simulink model "dc_microgrid"  (R2014a)
settings: Solver=ode45  StartTime=0.0  StopTime=Tmax  RelTol=1e-3
values from neighbouring files (symbols this model uses):
  a1v1 = Pmc*a1xpi1    [parameters_dcmicrogrid.m]
  a1v2 = Pmc*a1xpi2    [parameters_dcmicrogrid.m]
  a1xmc1 = a3    [parameters_dcmicrogrid.m]
  a1xmc2 = a3    [parameters_dcmicrogrid.m]
  a1xpi1 = Imc*c3    [parameters_dcmicrogrid.m]
  a1xpi2 = Imc*c3    [parameters_dcmicrogrid.m]
  a2v1 = Pmc*a2xpi1    [parameters_dcmicrogrid.m]
  a2v2 = Pmc*a2xpi2    [parameters_dcmicrogrid.m]
  a2xmc1 = C(1,2)*P(1,1)*c1/Imax(1)    [parameters_dcmicrogrid.m]
  a2xmc2 = C(2,1)*P(2,2)*c1/Imax(2)    [parameters_dcmicrogrid.m]
  a2xpi1 = Imc*c2    [parameters_dcmicrogrid.m]
  a2xpi2 = Imc*c2    [parameters_dcmicrogrid.m]
  a3xmc1 = C(1,2)*P(1,1)*c1/Imax(1) + RD(1,1)*c1    [parameters_dcmicrogrid.m]
  a3xmc2 = C(1,2)*P(2,2)*c1/Imax(2) + RD(2,2)*c1    [parameters_dcmicrogrid.m]
  axi1 = C(1,2)*I(1,1)*c1/Imax(1)    [parameters_dcmicrogrid.m]
  axi2 = C(2,1)*I(2,2)*c1/Imax(2)    [parameters_dcmicrogrid.m]
  C1 = 2.2e-3    (= 0.0022)    [parameters_dcmicrogrid.m]
  C2 = 2.2e-3    (= 0.0022)    [parameters_dcmicrogrid.m]
  iL1_0 = 4.5    [parameters_dcmicrogrid.m]
  iL2_0 = 4.5    [parameters_dcmicrogrid.m]
  L1 = 2.65e-3    (= 0.00265)    [parameters_dcmicrogrid.m]
  L2 = 2.65e-3    (= 0.00265)    [parameters_dcmicrogrid.m]
  R1 = 20    [parameters_dcmicrogrid.m]
  R2 = 20    [parameters_dcmicrogrid.m]
  Req = R1*R2/(R1+R2)    (= 10)    [parameters_dcmicrogrid.m]
  rL1 = 520e-3    (= 0.52)    [parameters_dcmicrogrid.m]
  rL2 = 520e-3    (= 0.52)    [parameters_dcmicrogrid.m]
  rs1 = 200e-3    (= 0.2)    [parameters_dcmicrogrid.m]
  rs2 = 200e-3    (= 0.2)    [parameters_dcmicrogrid.m]
  T1 = 1/Fs    (= 6.66666666667e-05)    [parameters_dcmicrogrid.m]
  T2 = 1/Fs    (= 6.66666666667e-05)    [parameters_dcmicrogrid.m]
  t_0 = 0    [parameters_dcmicrogrid.m]
  vC1_0 = 48.02    [parameters_dcmicrogrid.m]
  vC2_0 = 48.02    [parameters_dcmicrogrid.m]
  Vin1 = Vin(1)    [parameters_dcmicrogrid.m]
  Vin2 = Vin(2)    [parameters_dcmicrogrid.m]
  Vref1 = Vref(1)    [parameters_dcmicrogrid.m]
  Vref2 = Vref(2)    [parameters_dcmicrogrid.m]
  xi1_0 = 0.01915    [parameters_dcmicrogrid.m]
  xi2_0 = 0.01915    [parameters_dcmicrogrid.m]
  xmc1_0 = 2.401    [parameters_dcmicrogrid.m]
  xmc2_0 = 2.401    [parameters_dcmicrogrid.m]
  xpi1_0 = 0.51    [parameters_dcmicrogrid.m]
  xpi2_0 = 0.51    [parameters_dcmicrogrid.m]
  xpu1_0 = 0.01275    [parameters_dcmicrogrid.m]
  xpu2_0 = 0.01275    [parameters_dcmicrogrid.m]
  xvo1_0 = 0.0103    [parameters_dcmicrogrid.m]
  xvo2_0 = 0.0103    [parameters_dcmicrogrid.m]
undefined symbols (not defined in the file or in its folder): a1, a2, b1, b2, c1, c2, d1, d2
settings Model: Creator=OmarAli  LastModifiedBy=OmarAli
settings DataIOCC: LimitDataPoints=off
settings DebuggingCC: MergeDetectMultiDrivingBlocksExec=error  FrameProcessingCompatibilityMsg=error

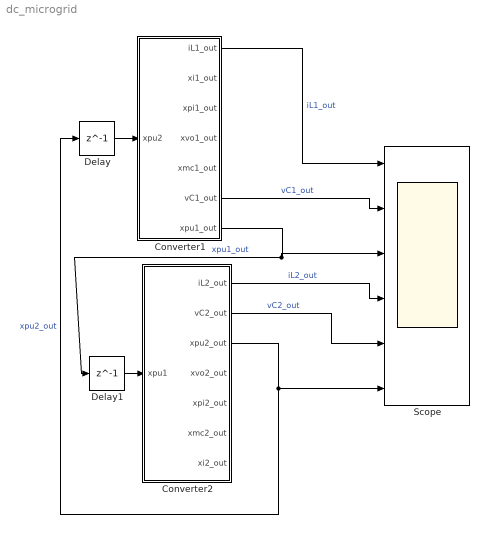
== system dc_microgrid ==
  Converter1 : Stateflow chart  TreatAsAtomicUnit=on
  Converter2 : Stateflow chart  TreatAsAtomicUnit=on
  Delay : Delay  DelayLength=1  InitialCondition=0  SampleTime=1/60000
  Delay1 : Delay  DelayLength=1  InitialCondition=0  SampleTime=1/60000
  Scope : Scope  NumInputPorts=6
      settings: ShowLegends=on  YMin=-5~-5~-5~-5~-5~-5  YMax=5~5~5~5~5~5
  wires:
  Converter1/7(xpu1_out) -> Scope/3, Delay1/1  "xpu1_out"
  Converter2/3(xpu2_out) -> Scope/6, Delay/1  "xpu2_out"
  Delay/1 -> Converter1/1(xpu2)
  Delay1/1 -> Converter2/1(xpu1)
  Converter1/1(iL1_out) -> Scope/1  "iL1_out"
  Converter1/6(vC1_out) -> Scope/2  "vC1_out"
  Converter2/1(iL2_out) -> Scope/4  "iL2_out"
  Converter2/2(vC2_out) -> Scope/5  "vC2_out"

== stateflow chart dc_microgrid/Converter2 ==
  settings: updateMethod=CONTINUOUS
  state close2
    du:
    iL2_dot = (1/L2)*(-1*(rs2+rL2)*iL2+Vin2 - vC2);
    vC2_dot = (1/C2)*(iL2 - vC2/Req);
    xpu2_dot = a1*xpu2 + b1*iL2;
    xi2_dot = axi2*(xpu1 - xpu2);
    xmc2_dot = a1xmc2*xmc2 + a2xmc2*xpu1 - a3xmc2*xpu2 + xi2+ Vref2;
    xvo2_dot = a2*xvo2 + b2*vC2;
    xpi2_dot = a1xpi2*xmc2 - a2xpi2*xvo2;
    t_dot = 1;
    iL2_out = iL2;
    vC2_out = vC2;
    xpu2_out = xpu2;
    xi2_out = xi2;
    xmc2_out =xmc2;
    xvo2_out = xvo2;
    xpi2_out = xpi2;
  state open2
    du:
    iL2_dot = (1/L2)*(-rL2*iL2 - vC2);
    vC2_dot = (1/C2)*(iL2 - vC2/Req);
    xpu2_dot = a1*xpu2 + b1*iL2;
    xi2_dot = axi2*(xpu1 - xpu2);
    xmc2_dot = a1xmc2*xmc2 + a2xmc2*xpu1 - a3xmc2*xpu2 + xi2+ Vref2;
    xvo2_dot = a2*xvo2 + b2*vC2;
    xpi2_dot = a1xpi2*xmc2 - a2xpi2*xvo2;
    t_dot = 1;
    iL2_out = iL2;
    vC2_out = vC2;
    xpu2_out = xpu2;
    xi2_out = xi2;
    xmc2_out =xmc2;
    xvo2_out = xvo2;
    xpi2_out = xpi2;
  state dcm2
    du:
    iL2_dot = 0;
    vC2_dot = - vC2/(Req*C2);
    xpu2_dot = a1*xpu2 + b1*iL2;
    xi2_dot = axi2*(xpu1 - xpu2);
    xmc2_dot = a1xmc2*xmc2 + a2xmc2*xpu1 - a3xmc2*xpu2 + xi2+ Vref2;
    xvo2_dot = a2*xvo2 + b2*vC2;
    xpi2_dot = a1xpi2*xmc2 - a2xpi2*xvo2;
    t_dot = 1;
    iL2_out = iL2;
    vC2_out = vC2;
    xpu2_out = xpu2;
    xi2_out = xi2;
    xmc2_out =xmc2;
    xvo2_out = xvo2;
    xpi2_out = xpi2;
  (default) -> close2 : {iL2 = iL2_0;
      | vC2 = vC2_0;
      | xpu2 = xpu2_0;
      | xi2 = xi2_0;
      | xmc2 = xmc2_0;
      | xvo2 = xvo2_0;
      | xpi2 = xpi2_0;
      | t = t_0;}
  close2 -> open2 : [(a1v2*xmc2 - a2v2*xvo2 + xpi2) -  t/T2<= 0]
  open2 -> close2 [order 2] : [t >= T2]
      | {t = 0;}
  dcm2 -> close2 : [t >= T2]
      | {t = 0;}
  open2 -> dcm2 [order 1] : [iL2 <= 0]
  data: rs2 parameter double; Vref2 parameter double; Vin2 parameter double; rL2 parameter double; iL2_out output double; t local; iL2 local; vC2 local; xi2 local; xvo2 local; xpu2 local; xmc2 local; xpi2 local; T2 parameter double; L2 parameter double; C2 parameter double; R2 parameter double; vC2_out output double; xpu2_out output double; xvo2_out output double; xpi2_out output double; xmc2_out output double; xi2_out output double; xpu1 input double; a1 parameter double; a2 parameter double; b1 parameter double; b2 parameter double; c1 parameter double; c2 parameter double; d1 parameter double; d2 parameter double; axi2 parameter double; a1xmc2 parameter double; a2xmc2 parameter double; a3xmc2 parameter double; a1xpi2 parameter double; a2xpi2 parameter double; a1v2 parameter double; a2v2 parameter double; Req parameter double; iL2_0 parameter; t_0 parameter; xpu2_0 parameter; xmc2_0 parameter; xvo2_0 parameter; xpi2_0 parameter; vC2_0 parameter; xi2_0 parameter
  data t settings: updateMethod=SF_CONTINUOUS_TIME_DATA
  data iL2 settings: updateMethod=SF_CONTINUOUS_TIME_DATA
  data vC2 settings: updateMethod=SF_CONTINUOUS_TIME_DATA
  data xi2 settings: updateMethod=SF_CONTINUOUS_TIME_DATA
  data xvo2 settings: updateMethod=SF_CONTINUOUS_TIME_DATA
  data xpu2 settings: updateMethod=SF_CONTINUOUS_TIME_DATA
  data xmc2 settings: updateMethod=SF_CONTINUOUS_TIME_DATA
  data xpi2 settings: updateMethod=SF_CONTINUOUS_TIME_DATA

== stateflow chart dc_microgrid/Converter1 ==
  settings: updateMethod=CONTINUOUS
  state close1
    du:
    iL1_dot = (1/L1)*(-1*(rs1+rL1)*iL1+Vin1 - vC1);
    vC1_dot = (1/C1)*(iL1 - vC1/Req);
    xpu1_dot = a1*xpu1 + b1*iL1;
    xi1_dot = axi1*(xpu2 - xpu1);
    xmc1_dot = a1xmc1*xmc1 + a2xmc1*xpu2  - a3xmc1*xpu1 + xi1+ Vref1;
    xvo1_dot = a2*xvo1 + b2*vC1;
    xpi1_dot = a1xpi1*xmc1 - a2xpi1*xvo1;
    t_dot = 1;
    iL1_out = iL1;
    vC1_out = vC1;
    xpu1_out = xpu1;
    xi1_out = xi1;
    xmc1_out =xmc1;
    xvo1_out = xvo1;
    xpi1_out = xpi1;
  state open1
    du:
    iL1_dot = (1/L1)*(-rL1*iL1 - vC1);
    vC1_dot = (1/C1)*(iL1 - vC1/Req);
    xpu1_dot = a1*xpu1 + b1*iL1;
    xi1_dot = axi1*(xpu2 - xpu1);
    xmc1_dot = a1xmc1*xmc1 + a2xmc1*xpu2  - a3xmc1*xpu1 + xi1+ Vref1;
    xvo1_dot = a2*xvo1 + b2*vC1;
    xpi1_dot = a1xpi1*xmc1 - a2xpi1*xvo1;
    t_dot = 1;
    iL1_out = iL1;
    vC1_out = vC1;
    xpu1_out = xpu1;
    xi1_out = xi1;
    xmc1_out =xmc1;
    xvo1_out = xvo1;
    xpi1_out = xpi1;
  state dcm1
    du:
    iL1_dot = 0;
    vC1_dot = - vC1/(Req*C1);
    xpu1_dot = a1*xpu1 + b1*iL1;
    xi1_dot = axi1*(xpu2 - xpu1);
    xmc1_dot = a1xmc1*xmc1 + a2xmc1*xpu2  - a3xmc1*xpu1 + xi1+ Vref1;
    xvo1_dot = a2*xvo1 + b2*vC1;
    xpi1_dot = a1xpi1*xmc1 - a2xpi1*xvo1;
    t_dot = 1;
    iL1_out = iL1;
    vC1_out = vC1;
    xpu1_out = xpu1;
    xi1_out = xi1;
    xmc1_out =xmc1;
    xvo1_out = xvo1;
    xpi1_out = xpi1;
  (default) -> close1 : {iL1 = iL1_0;
      | vC1 = vC1_0;
      | xpu1 = xpu1_0;
      | xi1 = xi1_0;
      | xmc1 = xmc1_0;
      | xvo1 = xvo1_0;
      | xpi1 = xpi1_0;
      | t = t_0;}
  close1 -> open1 : [(a1v1*xmc1 - a2v1*xvo1 + xpi1) -  t/T1 <= 0]
  open1 -> close1 [order 2] : [t >= T1]
      | {t = 0;}
  dcm1 -> close1 : [t >= T1]
      | {t = 0;}
  open1 -> dcm1 [order 1] : [iL1 <= 0]
  data: rL1 parameter double; Vin1 parameter double; rs1 parameter double; Vref1 parameter double; iL1_out output double; xpu1 local; iL1 local; xmc1 local; vC1 local; xpi1 local; xvo1 local; xi1 local; t local; C1 parameter double; R1 parameter double; L1 parameter double; T1 parameter double; xi1_out output double; xpi1_out output double; xvo1_out output double; xmc1_out output double; vC1_out output double; xpu1_out output double; xpu2 input double; a1 parameter double; a2 parameter double; b1 parameter double; b2 parameter double; c1 parameter double; c2 parameter double; d1 parameter double; d2 parameter double; axi1 parameter double; a1xmc1 parameter double; a2xmc1 parameter double; a3xmc1 parameter double; a1xpi1 parameter double; a2xpi1 parameter double; a1v1 parameter double; a2v1 parameter double; Req parameter double; xvo1_0 parameter; xpi1_0 parameter; xmc1_0 parameter; xi1_0 parameter; iL1_0 parameter; vC1_0 parameter; xpu1_0 parameter; t_0 parameter
  data xpu1 settings: updateMethod=SF_CONTINUOUS_TIME_DATA
  data iL1 settings: updateMethod=SF_CONTINUOUS_TIME_DATA
  data xmc1 settings: updateMethod=SF_CONTINUOUS_TIME_DATA
  data vC1 settings: updateMethod=SF_CONTINUOUS_TIME_DATA
  data xpi1 settings: updateMethod=SF_CONTINUOUS_TIME_DATA
  data xvo1 settings: updateMethod=SF_CONTINUOUS_TIME_DATA
  data xi1 settings: updateMethod=SF_CONTINUOUS_TIME_DATA
  data t settings: updateMethod=SF_CONTINUOUS_TIME_DATA
